simulink model "NE_3link_flexjoint_sim"  (R2020a)
settings: Solver=ode45  StartTime=0.0  StopTime=T  FixedStep=0.1  MaxStep=0.05  RelTol=1e-3
values from neighbouring files (symbols this model uses):
  bl = [0.2;0.2;0.2]    [simscape_NE_comparison.m]    (also in simscape_NE_flexjoint_comparison.m; simscape_example.m; simscape_flexjoint_example.m)
  bm = [0.03;0.03;0.03]    [simscape_NE_flexjoint_comparison.m]    (also in simscape_flexjoint_example.m)
  c = [[0.01;-0.05;-0.14],[0.03;0.045;-0.01],[-0.02;-0.01;0.13]]    [simscape_NE_comparison.m]    (also in simscape_NE_flexjoint_comparison.m; simscape_example.m; simscape_flexjoint_example.m)
  g = [0;0;-9.81]    [simscape_NE_comparison.m]    (also in simscape_NE_flexjoint_comparison.m; simscape_example.m; simscape_flexjoint_example.m)
  H = [[0;0;1],[0;1;0],[0;0;1]]    [simscape_NE_comparison.m]    (also in simscape_NE_flexjoint_comparison.m; simscape_example.m; simscape_flexjoint_example.m)
  Im = [0.4; 0.35; 0.28]    [simscape_NE_flexjoint_comparison.m]    (also in simscape_flexjoint_example.m)
  Ip = zeros(3,3,3)    [simscape_NE_comparison.m]    (also in simscape_NE_flexjoint_comparison.m)
  K = [50; 20; 15]    [simscape_NE_flexjoint_comparison.m]    (also in simscape_flexjoint_example.m)
  m = [3; 1.1; 2.4]    [simscape_NE_comparison.m]    (also in simscape_NE_flexjoint_comparison.m; simscape_example.m; simscape_flexjoint_example.m)
  N = [5; 3.3; 2.1]    [simscape_NE_flexjoint_comparison.m]    (also in simscape_flexjoint_example.m)
  P = [d1*z0, zeros(3,1), d2*y0, d3*z0]    [simscape_NE_comparison.m]    (also in simscape_NE_flexjoint_comparison.m; simscape_example.m; simscape_flexjoint_example.m)
  q0 = [0.3;-0.1;-.21]    [simscape_NE_comparison.m]    (also in simscape_NE_flexjoint_comparison.m = [0.5;-0.22;0.06]; simscape_example.m = [0;0;0]; simscape_flexjoint_example.m = [0;0;0])
  qdot0 = [0.03;0.004;-0.1]    [simscape_NE_comparison.m]    (also in simscape_NE_flexjoint_comparison.m = [0.01;0.02;-0.015]; simscape_example.m = [0;0;0]; simscape_flexjoint_example.m = [0;0;0])
  qm0 = N.*q0    [simscape_NE_flexjoint_comparison.m]    (also in simscape_flexjoint_example.m)
  qmdot0 = N.*qdot0    [simscape_NE_flexjoint_comparison.m]    (also in simscape_flexjoint_example.m)
  taustep = [3;-3;2]    [simscape_NE_comparison.m]    (also in simscape_NE_flexjoint_comparison.m = [1;-1.4;0.7]; simscape_example.m = [0;0;0]; simscape_flexjoint_example.m = [0;0;0])
settings Model: Creator=davidcarabis  LastModifiedBy=davidcarabis
settings DataIOCC: ReturnWorkspaceOutputs=off
settings DebuggingCC: ArithmeticOperatorsInVariantConditions=warning
settings SFSimCC: CustomCodeUndefinedFunction=UseInterfaceOnly

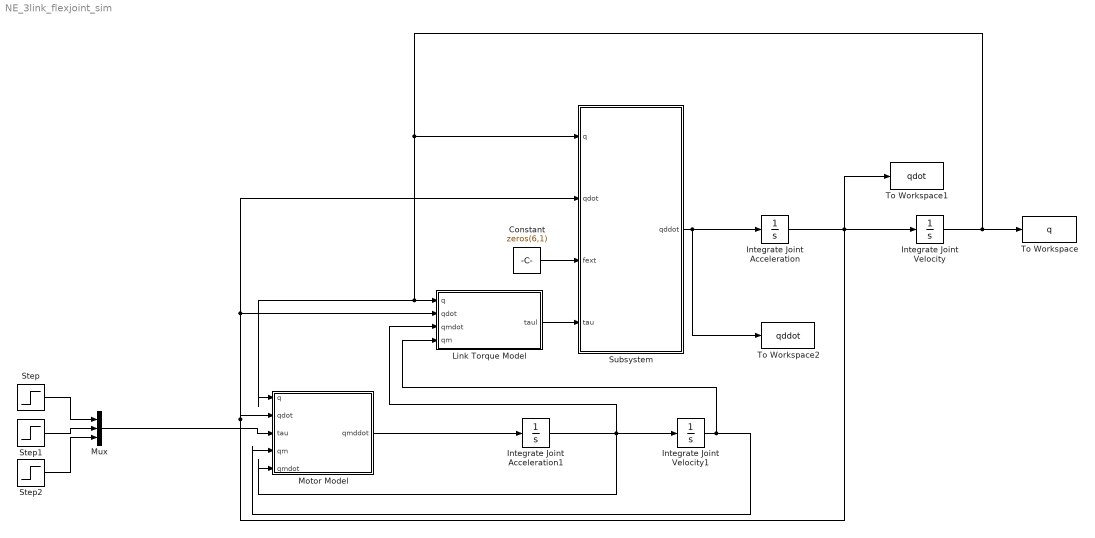
== system NE_3link_flexjoint_sim ==
  Constant : Constant  Value=zeros(6,1)
  Integrate Joint Acceleration : Integrator  InitialCondition=qdot0
  Integrate Joint Acceleration1 : Integrator  InitialCondition=qmdot0
  Integrate Joint Velocity : Integrator  InitialCondition=q0
  Integrate Joint Velocity1 : Integrator  InitialCondition=qm0
  Link Torque Model : Subsystem  mask{b=bl, K=K, N=N}
      mask prompts: b "Link Friction"; K "Spring Constants"; N "Gear Ratios"
  Motor Model : Subsystem  mask{bl=bl, K=K, N=N, Im=Im, bm=bm}
      mask prompts: bl "Link Friction"; K "Spring Constants"; N "Gear Ratios"; Im "Motor Inertias"; bm "Motor Damping"
  Mux : Mux  Inputs=3
  Step : Step  Time=0.5  Before=taustep(1)  After=0  SampleTime=0
  Step1 : Step  Time=0.5  Before=taustep(2)  After=0  SampleTime=0
  Step2 : Step  Time=0.5  Before=taustep(3)  After=0  SampleTime=0
  Subsystem : Subsystem  mask{h=H, p=P, m=m, c=c, I=Ip, V0=zeros(6,1), A0=[zeros(3,1);-g]}
      mask prompts: h "Rotation Axes"; p "Joint Offsets"; m "Link Masses"; c "Link COMs"; I "Link Inertias"
  To Workspace : ToWorkspace  VariableName=q  SampleTime=-1
  To Workspace1 : ToWorkspace  VariableName=qdot  SampleTime=-1
  To Workspace2 : ToWorkspace  VariableName=qddot  SampleTime=-1
  wires:
  Constant/1 -> Subsystem/3(fext)
  Link Torque Model/1(taul) -> Subsystem/4(tau)
  Subsystem/1(qddot) -> To Workspace2/1, Integrate Joint Acceleration/1
  Integrate Joint Acceleration/1 -> Motor Model/2(qdot), Link Torque Model/2(qdot), Subsystem/2(qdot), Integrate Joint Velocity/1, To Workspace1/1
  Step/1 -> Mux/1
  Step1/1 -> Mux/2
  Step2/1 -> Mux/3
  Integrate Joint Acceleration1/1 -> Motor Model/5(qmdot), Link Torque Model/3(qmdot), Integrate Joint Velocity1/1
  Integrate Joint Velocity1/1 -> Motor Model/4(qm), Link Torque Model/4(qm)
  Motor Model/1(qmddot) -> Integrate Joint Acceleration1/1
  Integrate Joint Velocity/1 -> To Workspace/1, Motor Model/1(q), Link Torque Model/1(q), Subsystem/1(q)
  Mux/1 -> Motor Model/3(tau)

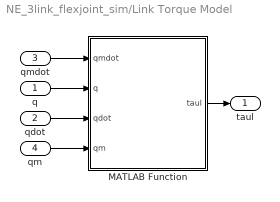
== system NE_3link_flexjoint_sim/Link Torque Model ==
  q : Inport
  qdot : Inport  Port=2
  qmdot : Inport  Port=3
  qm : Inport  Port=4
  MATLAB Function : MATLAB Function  TreatAsAtomicUnit=on
  taul : Outport  VectorParamsAs1DForOutWhenUnconnected=off
  wires:
  MATLAB Function/1(taul) -> taul/1
  q/1 -> MATLAB Function/2(q)
  qdot/1 -> MATLAB Function/3(qdot)
  qm/1 -> MATLAB Function/4(qm)
  qmdot/1 -> MATLAB Function/1(qmdot)

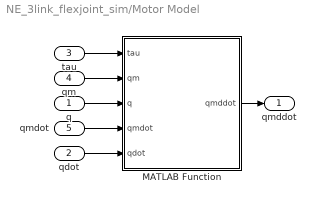
== system NE_3link_flexjoint_sim/Motor Model ==
  q : Inport
  qdot : Inport  Port=2
  tau : Inport  Port=3
  qm : Inport  Port=4
  qmdot : Inport  Port=5
  MATLAB Function : MATLAB Function  TreatAsAtomicUnit=on
  qmddot : Outport  VectorParamsAs1DForOutWhenUnconnected=off
  wires:
  MATLAB Function/1(qmddot) -> qmddot/1
  tau/1 -> MATLAB Function/1(tau)
  q/1 -> MATLAB Function/3(q)
  qm/1 -> MATLAB Function/2(qm)
  qdot/1 -> MATLAB Function/5(qdot)
  qmdot/1 -> MATLAB Function/4(qmdot)

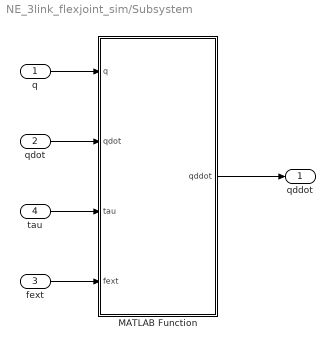
== system NE_3link_flexjoint_sim/Subsystem ==
  q : Inport
  qdot : Inport  Port=2
  fext : Inport  Port=3
  tau : Inport  Port=4
  MATLAB Function : MATLAB Function  TreatAsAtomicUnit=on
  qddot : Outport  VectorParamsAs1DForOutWhenUnconnected=off
  wires:
  tau/1 -> MATLAB Function/3(tau)
  MATLAB Function/1(qddot) -> qddot/1
  qdot/1 -> MATLAB Function/2(qdot)
  fext/1 -> MATLAB Function/4(fext)
  q/1 -> MATLAB Function/1(q)

== matlab function NE_3link_flexjoint_sim/Link Torque Model/MATLAB Function ==
  data: K parameter; qmdot input; q input; taul output; qdot input; qm input; bl parameter; N parameter
function taul = friction(K,qmdot,q,qdot, qm, bl, N)

taul = K.*(1./N.*qm - q) + bl.*(1./N.*qmdot - qdot);

== matlab function NE_3link_flexjoint_sim/Subsystem/MATLAB Function ==
  data: q input; qdot input; tau input; qddot output; fext input; h parameter; p parameter; I parameter; m parameter; c parameter; V0 parameter; A0 parameter
function qddot  = NEalgorithm(q,qdot,tau,fext,h,p,I,m,c,V0,A0)


% Implement Newton Euler Algorithm

% Generate H, PHI block matrices (assumes all rotational joints)
H = blkdiag([h(:,1);zeros(3,1)],[h(:,2);zeros(3,1)],[h(:,3);zeros(3,1)]);

PHI = phi_gen(q,h,p);

% Forward sweep to compute V,a,b,M

V = zeros(6,3);
Vtemp = V0;
Vprev = V0;
a = zeros(6,3);
b = zeros(6,3);
M = zeros(6,6,3);

for k = 1:3
    PHI_TEMP = PHI((6*k-5):6*k,(6*k-5):6*k);
    Htemp = H((6*k-5):6*k,k);
    Vtemp = PHI_TEMP*Vtemp + Htemp*qdot(k);
    V(:,k) = Vtemp;
    
    R = rot(h(:,k),q(k));
    
    a(:,k) = [hat(R'*Vprev(1:3))*(Vtemp(1:3));...
        R'*hat(Vprev(1:3))*(hat(Vprev(1:3))*p(:,k))];
    Vprev = Vtemp;
    
    b(:,k) = [hat(Vtemp(1:3))*I(:,:,k)*Vtemp(1:3); ...
        m(k)*hat(Vtemp(1:3))*hat(Vtemp(1:3))*c(:,k)];
    
    M(:,:,k) = [I(:,:,k) m(k)*hat(c(:,k));...
        -m(k)*hat(c(:,k)) m(k)*eye(3)];
    
end

% Backwards sweep for P, B

P = zeros(6,6,3);
B = zeros(6,6,3);

% Handle boundary condition first
PHIT3 = [eye(3) zeros(3); -eye(3)*hat(p(:,3)) eye(3)];
P(:,:,3) = M(:,:,3);
B(:,3) = PHIT3'*fext + b(:,3);

for k = 2:-1:1
    PHI_TEMP = PHI((6*k+1):(6*k+6),(6*k + 1):(6*k+6));
    Htemp = H((6*k+1):(6*k+6),k+1);
    P(:,:,k) = M(:,:,k) + PHI_TEMP'*P(:,:,k+1)*PHI_TEMP - ...
        (PHI_TEMP'*P(:,:,k+1)*Htemp*Htemp'*P(:,:,k+1)*PHI_TEMP)/...
        (Htemp'*P(:,:,k+1)*Htemp);
    
    B(:,k) = PHI_TEMP'*(P(:,:,k+1)*a(:,k+1) + B(:,k+1)) + b(:,k) + ...
        (PHI_TEMP'*P(:,:,k+1)*Htemp*(tau(k+1) - Htemp'*...
        (P(:,:,k+1)*a(:,k+1) + B(:,k+1))))/(Htemp'*P(:,:,k+1)*Htemp);
end

% Sweep Forward for qddot, A, f

qddot = zeros(3,1);
Atemp = A0;
f = zeros(6,3);

for k = 1:3
    atemp = a(:,k);
    PHI_TEMP = PHI((6*(k) - 5):(6*(k)),(6*(k) - 5):(6*(k)));
    Htemp = H((6*(k) - 5):(6*(k)),k);
    qddot(k) = (tau(k) - Htemp'*P(:,:,k)*PHI_TEMP*Atemp - Htemp'*...
        (P(:,:,k)*atemp + B(:,k)))/(Htemp'*P(:,:,k)*Htemp);
    
    Atemp = PHI_TEMP*Atemp + Htemp*qddot(k) + a(:,k);
    f(:,k) = P(:,:,k)*Atemp + B(:,k);
end

== matlab function NE_3link_flexjoint_sim/Motor Model/MATLAB Function ==
  data: tau input; K parameter; N parameter; bl parameter; qm input; q input; qmdot input; qmddot output; qdot input; Im parameter; bm parameter
function qmddot = friction(tau, K, N,bl, qm, q, qmdot, qdot, Im, bm)

qmddot = (tau - qmdot.*bm + K./N.*(q - 1./N.*qm) + bl./N.*(qdot - 1./N.*qmdot))./Im;
